simulink model "electrico_sim"  (R2022b)
settings: Solver=VariableStepAuto  StartTime=0.0  StopTime=10.0  RelTol=1e-3
values from neighbouring files (symbols this model uses):
  c = 1    [electrico.m]
  l = 1    [electrico.m]    (also in electromecanico.m = 0.5)
settings Model: Creator=Fran  LastModifiedBy=Fran

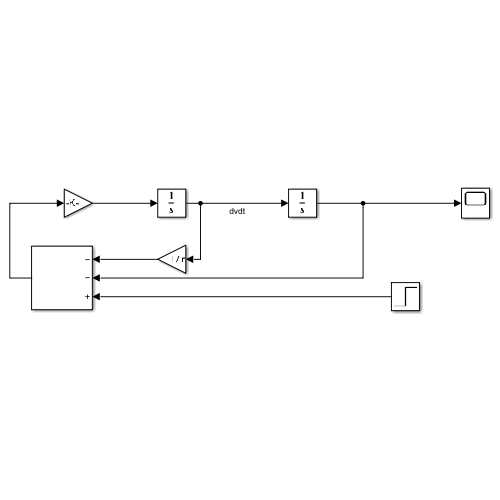
[thumbnail: Simulink's stored preview of the top-level diagram]
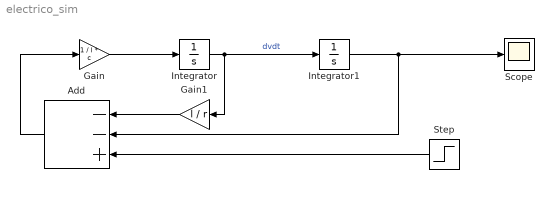
== system electrico_sim ==
  Add : Sum  Inputs=--+
  Gain : Gain  Gain=1 / l * c
  Gain1 : Gain  Gain=l / r
  Integrator : Integrator
  Integrator1 : Integrator
  Scope : Scope
  Step : Step  SampleTime=0
  wires:
  Integrator/1 -> Gain1/1, Integrator1/1  "dvdt"
  Gain/1 -> Integrator/1
  Gain1/1 -> Add/1
  Integrator1/1 -> Scope/1, Add/2
  Step/1 -> Add/3
  Add/1 -> Gain/1
